simulink model "hf_throwsimulink"  (R2022a)
settings: Solver=VariableStepAuto  StartTime=0.0  StopTime=10  FixedStep=.01  RelTol=1e-7  EnableMultiTasking=on
undefined symbols (not defined in the file or in its folder): vw
settings Model: Creator=SLE  LastModifiedBy=ASUS
settings SolverCC: AlgebraicLoopSolver=TrustRegion
settings DataIOCC: Decimation=4  SaveFormat=Array  SignalLoggingSaveFormat=ModelDataLogs  SignalLogging=off  SaveTime=off  ReturnWorkspaceOutputs=off
settings OptimizationCC: ExpressionDepthLimit=2147483647  LifeSpan=inf
settings DebuggingCC: UnderspecifiedInitializationDetection=Classic  MergeDetectMultiDrivingBlocksExec=none  SolverPrmCheckMsg=warning  UnconnectedInputMsg=warning  UnconnectedOutputMsg=warning  UnconnectedLineMsg=warning  StateNameClashWarn=warning  SFUnexpectedBacktrackingDiag=warning  SFNoUnconditionalDefaultTransitionDiag=warning  SFExecutionAtInitializationDiag=none  SFMachineParentedDataDiag=warning  ArithmeticOperatorsInVariantConditions=warning
settings HardwareCC: ProdBitPerPointer=32  ProdBitPerSizeT=32  ProdBitPerPtrDiffT=32  ProdLargestAtomicFloat=None  ProdIntDivRoundTo=Undefined  ProdEndianess=Unspecified  ProdWordSize=32  ProdHWDeviceType=32-bit Generic
settings ModelReferenceCC: PropagateSignalLabelsOutOfModel=off
settings SFSimCC: SimUseLocalCustomCode=off  CustomCodeUndefinedFunction=UseInterfaceOnly  SimTargetLang=C++
settings RTWCC: GenCodeOnly=on  GenerateReport=on  TLCDebug=on  TLCAssert=on  RTWUseLocalCustomCode=off  RTWUseSimCustomCode=on  LaunchReport=on  TargetLang=C++
settings CodeAppCC: ForceParamTrailComments=on  StateflowObjectComments=on  UseSimReservedNames=on
settings GRTTargetCC: TargetLangStandard=C89/C90 (ANSI)  CombineOutputUpdateFcns=off  GRTInterface=on
settings ConfigComp: CovMetricSettings=dw  CovSaveCumulativeToWorkspaceVar=on  CovSaveSingleToWorkspaceVar=on  CovExternalEMLEnable=off

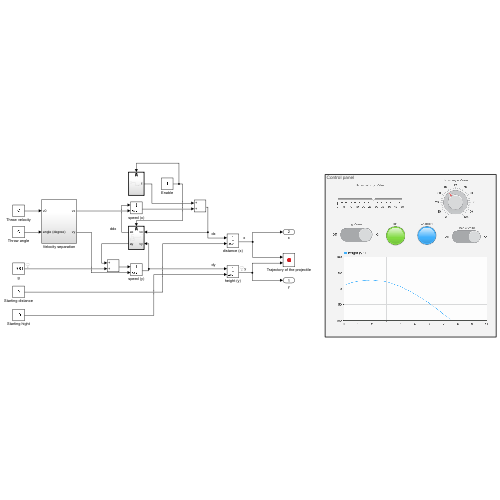
[thumbnail: Simulink's stored preview of the top-level diagram]
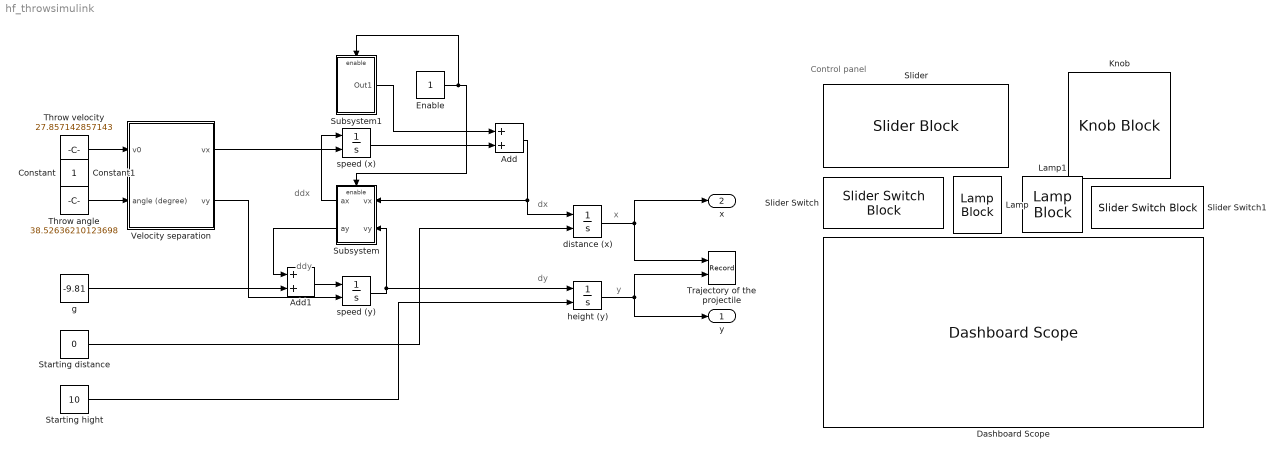
== system hf_throwsimulink ==
  note: Control panel
  note: dx
  note: x
  note: dy
  note: ddy
  note: y
  note: ddx
  Add : Sum
  Add1 : Sum
  Dashboard Scope : DashboardScope  Ymin=-100  Ymax=100  ScaleAtStop=off
  Enable : Constant
  Knob : KnobBlock
  Lamp : LampBlock
  Lamp1 : LampBlock
  Slider : SliderBlock  ScaleMax=50
  Slider Switch : SliderSwitchBlock
      settings: Values={{'Off', 'On'}, [0 -9.81]}
  Slider Switch1 : SliderSwitchBlock
      settings: Values={{'Off', 'On'}, [0 1]}
  Starting distance : Constant  Value=0
  Starting hight : Constant  Value=10
  Subsystem : Subsystem
  Subsystem1 : Subsystem
  Throw angle : Constant  Value=38.52636210123698
  "Throw velocity " : Constant  Value=27.857142857143
  Trajectory of the projectile : Record  FileSettingsInternal="{\"entries\":[{\"content\":{\"excelSettings\":{\"content\":{},\"type\":\"Streamout.ExcelSettings\"}},\"type\":\"Streamout.FileSettingStorage\",\"uuid\":\"ddf4c1e3-71ed-404d-9800-dd86dffaf740\"}],\"packageUris\":[\"http://schema.mathworks.com/mf0/streamout_blocks/R2020a\"],\"version\":\"1.0\"}"  Layout=[1 1]  SignalsInternal="{\"entries\":[{\"content\":{\"signals\":[{\"content\":{\"blockPath\":[\"throw_simulink/Trajectory of the projectile\"],\"channel\":[],\"dimensions\":[1],\"domain\":\"throw_simulink/Trajectory of the projectile\",\"lineColor\":\"#a2142f\",\"plots\":[1],\"port\":1,\"sid\":[\"\"],\"signalID\":5418,\"signalName\":\"distance (x)\"},\"type\":\"RecordBlkView.Signal\",\"uuid\":\"c7814d3a-2678-4566-b8b1-f51774df6c6e\"},{\"content\":{\"blockPath\":[\"throw_simulink/Trajectory of the projectile\"],\"channel\":[],\"dimensions\":[1],\"domain\":\"throw_simulink/Trajectory of the projectile\",\"lineColor\":\"#139fff\",\"plots\":[1],\"port\":2,\"sid\":[\"\"],\"signalID\":5422,\"signalName\":\"height (y)\"},\"type\":\"RecordBlkView.Signal\",\"uuid\":\"f15c709c-8669-4a07-b773-59e362a044ca\"}]},\"type\":\"RecordBlkView.InputSignals\",\"uuid\":\"c9012ba7-3407-452c-9598-9ee1c77c03bb\"}],\"packageUris\":[\"http://schema.mathworks.com/mf0/streamout_blocks/R2020a\"],\"version\":\"1.0\"}"  VisualizationBindings="{\"xyplotplugin\":{\"info\":[{\"series\":[{\"bindingParametersList\":[{\"parameter\":\"X-Axis\",\"signalID\":5418,\"signalName\":\"distance (x)\"},{\"parameter\":\"Y-Axis\",\"signalID\":5422,\"signalName\":\"height (y)\"}],\"seriesID\":35491}],\"subplotID\":1}]}}"  CompatibilityTag=XY  st=-1
  Velocity separation : Subsystem
  distance (x) : Integrator  InitialConditionSource=external
  g : Constant  Value=-9.81
  height (y) : Integrator  InitialConditionSource=external  InitialCondition=1
  speed (x) : Integrator  InitialConditionSource=external
  speed (y) : Integrator  InitialConditionSource=external  InitialCondition=25*sin(15*pi/180)
  y : Outport  VectorParamsAs1DForOutWhenUnconnected=off
  x : Outport  Port=2  VectorParamsAs1DForOutWhenUnconnected=off
  Constant : Constant  IOType=siggen
  Constant1 : Constant  IOType=siggen
  wires:
  speed (y)/1 -> Subsystem/2(vy), height (y)/1
  height (y)/1 -> y/1, Trajectory of the projectile/2
  speed (x)/1 -> Add/2
  distance (x)/1 -> Trajectory of the projectile/1, x/1
  Starting distance/1 -> distance (x)/2
  Starting hight/1 -> height (y)/2
  "Throw velocity "/1 -> Velocity separation/1(v0)
  Throw angle/1 -> Velocity separation/2(angle (degree))
  Velocity separation/1(vx) -> speed (x)/2
  Velocity separation/2(vy) -> speed (y)/2
  Add/1 -> Subsystem/1(vx), distance (x)/1
  Add1/1 -> speed (y)/1
  g/1 -> Add1/2
  Subsystem/1(ax) -> speed (x)/1
  Subsystem/2(ay) -> Add1/1
  Subsystem1/1(Out1) -> Add/1
  Enable/1 -> Subsystem1/Enable, Subsystem/Enable

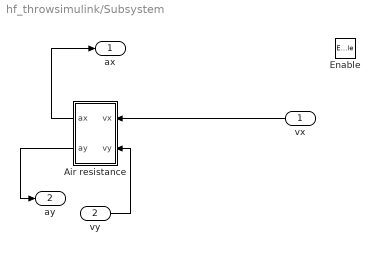
== system hf_throwsimulink/Subsystem ==
  vx : Inport
  vy : Inport  Port=2
  Enable : EnablePort
  Air resistance : Subsystem
  ax : Outport
  ay : Outport  Port=2
  wires:
  Air resistance/2(ay) -> ay/1
  vx/1 -> Air resistance/1(vx)
  vy/1 -> Air resistance/2(vy)
  Air resistance/1(ax) -> ax/1

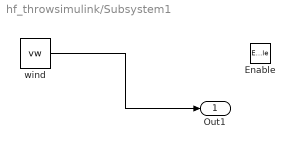
== system hf_throwsimulink/Subsystem1 ==
  Enable : EnablePort
  wind : Constant  InitFcn=vw = round(rand(1)*30-15,1);  Value=vw
  Out1 : Outport
  wires:
  wind/1 -> Out1/1

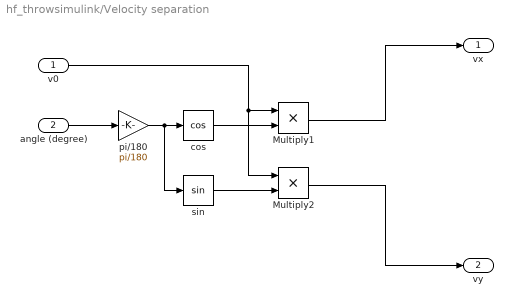
== system hf_throwsimulink/Velocity separation ==
  v0 : Inport
  angle (degree) : Inport  Port=2
  Multiply1 : Product
  Multiply2 : Product
  cos : Trigonometry  Operator=cos
  pi/180 : Gain  Gain=pi/180
  sin : Trigonometry
  vx : Outport  VectorParamsAs1DForOutWhenUnconnected=off
  vy : Outport  Port=2  VectorParamsAs1DForOutWhenUnconnected=off
  wires:
  Multiply1/1 -> vx/1
  sin/1 -> Multiply2/2
  angle (degree)/1 -> pi/180/1
  pi/180/1 -> cos/1, sin/1
  cos/1 -> Multiply1/2
  v0/1 -> Multiply2/1, Multiply1/1
  Multiply2/1 -> vy/1

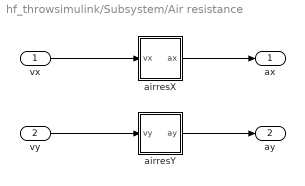
== system hf_throwsimulink/Subsystem/Air resistance ==
  vx : Inport
  vy : Inport  Port=2
  airresX : Subsystem
  airresY : Subsystem
  ax : Outport  VectorParamsAs1DForOutWhenUnconnected=off
  ay : Outport  Port=2  VectorParamsAs1DForOutWhenUnconnected=off
  wires:
  airresY/1(ay) -> ay/1
  vy/1 -> airresY/1(vy)
  vx/1 -> airresX/1(vx)
  airresX/1(ax) -> ax/1

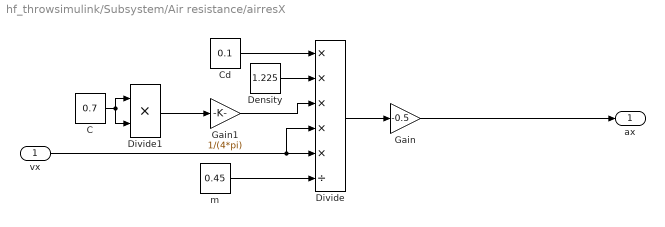
== system hf_throwsimulink/Subsystem/Air resistance/airresX ==
  vx : Inport
  C : Constant  Value=0.7
  Cd : Constant  Value=0.1
  Density : Constant  Value=1.225
  Divide : Product  Inputs=*****/
  Divide1 : Product  Inputs=**
  Gain : Gain  Gain=-0.5
  Gain1 : Gain  Gain=1/(4*pi)
  m : Constant  Value=0.45
  ax : Outport  VectorParamsAs1DForOutWhenUnconnected=off
  wires:
  C/1 -> Divide1/1, Divide1/2
  Gain1/1 -> Divide/3
  Divide1/1 -> Gain1/1
  Gain/1 -> ax/1
  vx/1 -> Divide/5, Divide/4
  m/1 -> Divide/6
  Density/1 -> Divide/2
  Cd/1 -> Divide/1
  Divide/1 -> Gain/1

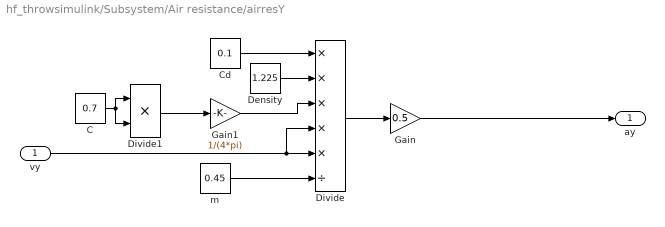
== system hf_throwsimulink/Subsystem/Air resistance/airresY ==
  vy : Inport
  C : Constant  Value=0.7
  Cd : Constant  Value=0.1
  Density : Constant  Value=1.225
  Divide : Product  Inputs=*****/
  Divide1 : Product  Inputs=**
  Gain : Gain  Gain=0.5
  Gain1 : Gain  Gain=1/(4*pi)
  m : Constant  Value=0.45
  ay : Outport  VectorParamsAs1DForOutWhenUnconnected=off
  wires:
  Divide/1 -> Gain/1
  Cd/1 -> Divide/1
  Density/1 -> Divide/2
  m/1 -> Divide/6
  vy/1 -> Divide/4, Divide/5
  Gain/1 -> ay/1
  Divide1/1 -> Gain1/1
  Gain1/1 -> Divide/3
  C/1 -> Divide1/2, Divide1/1
